simulink model "sampleModel1983"  (R2023a)
settings: Solver=VariableStepAuto  StartTime=0.0  StopTime=10.0  RelTol=1e-3
libraries: hdlsllib x7, simulink x2
settings Model: Creator=user1  LastModifiedBy=user1

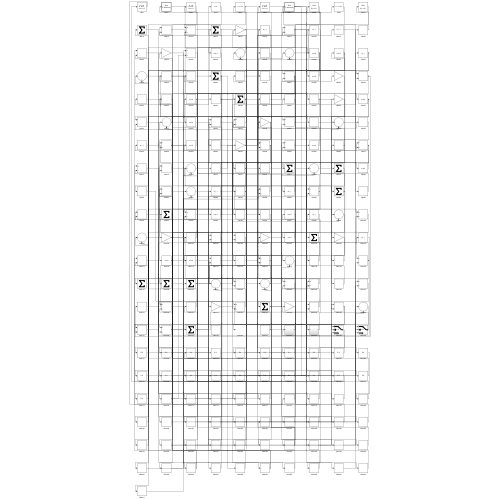
[thumbnail: Simulink's stored preview of the top-level diagram]
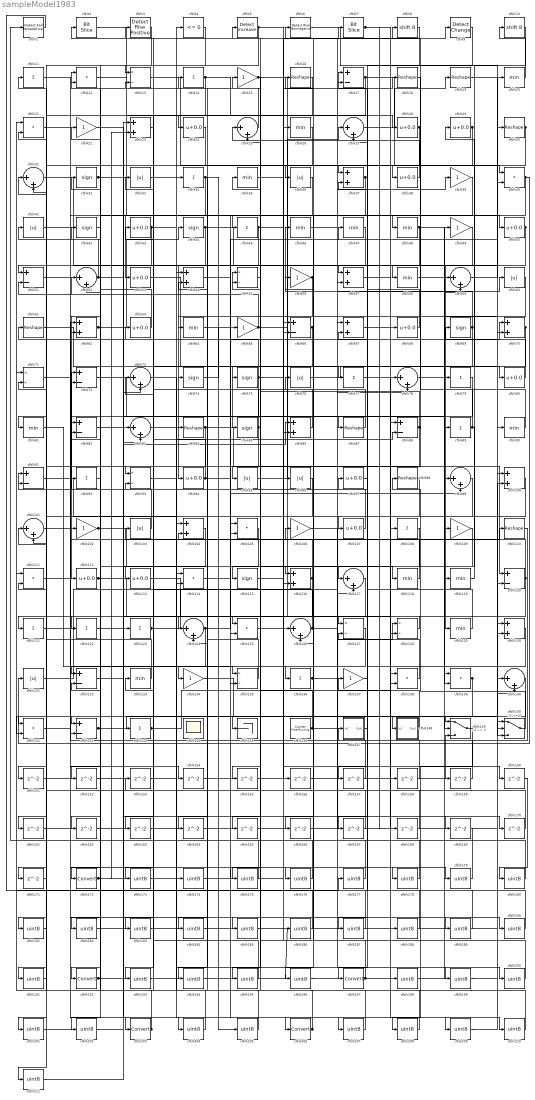
== system sampleModel1983 ==
  cfblk1 : hdlsllib/Logic and Bit Operations/Detect Fall Nonpositive  vinit=0  OutDataTypeStr=boolean
  cfblk10 : ArithShift  BitShiftNumber=8
  cfblk{23,37,54,57,62,67,70,86,100,104,116,130} (12 alike) : Sum
  cfblk{25,27,31,52,59,73,78,83,99,101,117,124,126,140} (14 alike) : Sum  Inputs=|++
  cfblk{15,22,39,49,56,65,102,106,109,134,137} (11 alike) : Gain
  cfblk{33,36,41,60,76,95..96,103,131} (9 alike) : Abs  SaturateOnIntegerOverflow=off
  cfblk{12,21,40,105,111,114,125,138..139,141} (10 alike) : DotProduct  OutDataTypeStr=Inherit: Inherit via internal rule
  cfblk{24,28..29,38,43,50,53,63,68,80,94,97,107,112..113} (15 alike) : Bias  Bias=0.0  SaturateOnIntegerOverflow=off
  cfblk{11,14,34,45,77,79,89,92,108,121..123,136,143} (14 alike) : Sum  Inputs=+
  cfblk{16,18..19,30,61,84,87,98,110} (9 alike) : Reshape
  cfblk{32,42,44,69,74..75,85,115} (8 alike) : Signum
  cfblk{20,26,35,46..48,58,64,81,90,118..119,129,133} (14 alike) : MinMax
  cfblk{17,51,66,72,82,88,91,120,132,142} (10 alike) : Sum  Inputs=+-
  cfblk{13,55,71,93,127..128,135} (7 alike) : Product  Inputs=*/  RndMeth=Zero  SaturateOnIntegerOverflow=on
  cfblk144 : Scope
      settings: Floating=on
  cfblk145 : Terminator
  cfblk146 : hdlsllib/Sources/Counter Free-Running  NumBits=16  tsamp=-1
  cfblk147 : Subsystem
      settings: LibrarySourceBlock=|
      | hdlsllib/Ports &
      | Subsystems/Subsystem
  cfblk148 : Subsystem
      settings: LibrarySourceBlock=|
      | hdlsllib/Ports &
      | Subsystems/Subsystem
  cfblk149 : Switch  SaturateOnIntegerOverflow=off  InputSameDT=off
  cfblk150 : Switch  SaturateOnIntegerOverflow=off  InputSameDT=off
  cfblk{151..171} (21 alike) : Delay  SampleTime=1
  cfblk{172,192,197,203,206} (5 alike) : DataTypeConversion  SaturateOnIntegerOverflow=off  RndMeth=Floor
  cfblk{173..191,193..196,198..202,204..205,207..211} (35 alike) : DataTypeConversion  OutDataTypeStr=uint8  SaturateOnIntegerOverflow=off  RndMeth=Floor
  cfblk2 : hdlsllib/Logic and Bit Operations/Bit Slice  lidx=7  ridx=0
  cfblk3 : hdlsllib/Logic and Bit Operations/Detect Rise Positive  vinit=0  OutDataTypeStr=boolean
  cfblk4 : hdlsllib/Logic and Bit Operations/Compare To Zero  relop=<=  OutDataTypeStr=boolean
  cfblk5 : simulink/Logic and Bit Operations/Detect Increase  vinit=0.0  OutDataTypeStr=boolean
      settings: LibrarySourceBlock=|
      | hdlsllib/Logic and Bit
      | Operations/Detect
      | Increase
  cfblk6 : hdlsllib/Logic and Bit Operations/Detect Rise Nonnegative  vinit=0  OutDataTypeStr=boolean
  cfblk7 : hdlsllib/Logic and Bit Operations/Bit Slice  lidx=7  ridx=0
  cfblk8 : ArithShift  BitShiftNumber=8
  cfblk9 : simulink/Logic and Bit Operations/Detect Change  vinit=0  OutDataTypeStr=boolean
      settings: LibrarySourceBlock=|
      | hdlsllib/Logic and Bit
      | Operations/Detect
      | Change
  wires:
  cfblk44/1 -> cfblk57/1, cfblk116/1, cfblk181/1
  cfblk33/1 -> cfblk34/1
  cfblk122/1 -> cfblk123/1
  cfblk25/1 -> cfblk12/1
  cfblk134/1 -> cfblk148/1(In1)
  cfblk38/1 -> cfblk25/1
  cfblk18/1 -> cfblk95/1
  cfblk95/1 -> cfblk27/1
  cfblk15/1 -> cfblk127/1, cfblk45/1
  cfblk4/1 -> cfblk172/1
  cfblk120/1 -> cfblk27/2, cfblk124/2
  cfblk116/1 -> cfblk3/1, cfblk201/1
  cfblk81/1 -> cfblk135/1
  cfblk86/1 -> cfblk76/1
  cfblk52/1 -> cfblk41/1, cfblk116/2
  cfblk50/1 -> cfblk94/1, cfblk139/2
  cfblk110/1 -> cfblk147/1(In1)
  cfblk74/1 -> cfblk65/1
  cfblk13/1 -> cfblk40/1
  cfblk40/1 -> cfblk131/1, cfblk59/1
  cfblk143/1 -> cfblk84/1, cfblk128/2
  cfblk8/1 -> cfblk107/1
  cfblk55/1 -> cfblk15/1
  cfblk62/1 -> cfblk44/1, cfblk86/2
  cfblk130/1 -> cfblk197/1
  cfblk42/1 -> cfblk112/1
  cfblk69/1 -> cfblk46/1, cfblk105/2
  cfblk66/1 -> cfblk163/1, cfblk164/1
  cfblk112/1 -> cfblk138/2, cfblk82/1
  cfblk36/1 -> cfblk53/1
  cfblk59/1 -> cfblk30/1
  cfblk65/1 -> cfblk20/1, cfblk8/1, cfblk51/2
  cfblk87/1 -> cfblk61/1
  cfblk3/1 -> cfblk81/1
  cfblk28/1 -> cfblk38/1, cfblk31/2, cfblk167/1
  cfblk71/1 -> cfblk203/1
  cfblk128/1 -> cfblk121/1
  cfblk94/1 -> cfblk43/1, cfblk70/1
  cfblk85/1 -> cfblk63/1, cfblk191/1
  cfblk9/1 -> cfblk37/1
  cfblk20/1 -> cfblk10/1
  cfblk68/1 -> cfblk17/1
  cfblk79/1 -> cfblk102/1
  cfblk103/1 -> cfblk11/1
  cfblk117/1 -> cfblk126/2
  cfblk118/1 -> cfblk16/1
  cfblk76/1 -> cfblk80/1
  cfblk58/1 -> cfblk129/1
  cfblk102/1 -> cfblk117/1, cfblk86/1
  cfblk131/1 -> cfblk26/1
  cfblk150/1 -> cfblk98/1
  cfblk105/1 -> cfblk115/1
  cfblk32/1 -> cfblk135/2, cfblk204/1
  cfblk56/1 -> cfblk74/1, cfblk75/1
  cfblk53/1 -> cfblk105/1
  cfblk114/1 -> cfblk47/1
  cfblk75/1 -> cfblk134/1, cfblk18/1, cfblk13/2
  cfblk133/1 -> cfblk91/1
  cfblk34/1 -> cfblk124/1, cfblk173/1, cfblk205/1
  cfblk78/1 -> cfblk89/1
  cfblk31/1 -> cfblk90/1
  cfblk17/1 -> cfblk40/2, cfblk141/1, cfblk170/1
  cfblk148/1(Out1) -> cfblk127/2
  cfblk147/1(Out1) -> cfblk37/2
  cfblk104/1 -> cfblk192/1
  cfblk39/1 -> cfblk142/1
  cfblk26/1 -> cfblk36/1
  cfblk12/1 -> cfblk108/1
  cfblk138/1 -> cfblk67/2
  cfblk124/1 -> cfblk142/2, cfblk99/2
  cfblk142/1 -> cfblk150/2, cfblk169/1
  cfblk82/1 -> cfblk125/1
  cfblk35/1 -> cfblk118/1
  cfblk126/1 -> cfblk60/1, cfblk33/1
  cfblk70/1 -> cfblk113/1, cfblk85/1
  cfblk48/1 -> cfblk132/1, cfblk70/2
  cfblk139/1 -> cfblk145/1, cfblk141/2
  cfblk41/1 -> cfblk58/1
  cfblk125/1 -> cfblk17/2
  cfblk107/1 -> cfblk72/1
  cfblk93/1 -> cfblk88/2
  cfblk43/1 -> cfblk48/1, cfblk211/1
  cfblk72/1 -> cfblk109/1
  cfblk132/1 -> cfblk143/1
  cfblk129/1 -> cfblk103/1
  cfblk108/1 -> cfblk136/1
  cfblk135/1 -> cfblk14/1
  cfblk47/1 -> cfblk64/1
  cfblk84/1 -> cfblk120/1, cfblk92/1
  cfblk14/1 -> cfblk28/1, cfblk193/1
  cfblk46/1 -> cfblk39/1
  cfblk6/1 -> cfblk150/3
  cfblk113/1 -> cfblk125/2
  cfblk64/1 -> cfblk149/1
  cfblk30/1 -> cfblk87/1, cfblk62/2
  cfblk90/1 -> cfblk7/1
  cfblk27/1 -> cfblk19/1
  cfblk11/1 -> cfblk50/1
  cfblk63/1 -> cfblk32/1
  cfblk16/1 -> cfblk24/1
  cfblk23/1 -> cfblk93/1
  cfblk88/1 -> cfblk55/1, cfblk162/1
  cfblk141/1 -> cfblk72/2
  cfblk100/1 -> cfblk122/1
  cfblk10/1 -> cfblk79/1
  cfblk29/1 -> cfblk51/1, cfblk155/1
  cfblk91/1 -> cfblk114/1
  cfblk54/1 -> cfblk206/1
  cfblk80/1 -> cfblk69/1
  cfblk5/1 -> cfblk66/2, cfblk13/1
  cfblk7/1 -> cfblk99/1, cfblk168/1, cfblk210/1
  cfblk89/1 -> cfblk119/1, cfblk2/1
  cfblk37/1 -> cfblk166/1, cfblk194/1, cfblk196/1
  cfblk61/1 -> cfblk77/1
  cfblk2/1 -> cfblk68/1
  cfblk146/1 -> cfblk149/2, cfblk25/2
  cfblk121/1 -> cfblk110/1
  cfblk45/1 -> cfblk160/1, cfblk161/1
  cfblk123/1 -> cfblk78/2, cfblk57/2
  cfblk119/1 -> cfblk29/1
  cfblk136/1 -> cfblk9/1, cfblk128/1
  cfblk19/1 -> cfblk100/1
  cfblk24/1 -> cfblk151/1
  cfblk151/1 -> cfblk114/2
  cfblk98/1 -> cfblk152/1
  cfblk51/1 -> cfblk154/1
  cfblk154/1 -> cfblk126/1
  cfblk155/1 -> cfblk149/3
  cfblk115/1 -> cfblk156/1
  cfblk97/1 -> cfblk157/1
  cfblk157/1 -> cfblk67/1
  cfblk57/1 -> cfblk158/1
  cfblk158/1 -> cfblk62/1
  cfblk159/1 -> cfblk88/1
  cfblk161/1 -> cfblk117/2
  cfblk162/1 -> cfblk59/2
  cfblk163/1 -> cfblk138/1
  cfblk164/1 -> cfblk120/2
  cfblk109/1 -> cfblk165/1
  cfblk165/1 -> cfblk78/1
  cfblk166/1 -> cfblk100/2
  cfblk167/1 -> cfblk52/2
  cfblk168/1 -> cfblk31/1
  cfblk169/1 -> cfblk1/1
  cfblk170/1 -> cfblk132/2
  cfblk96/1 -> cfblk171/1
  cfblk171/1 -> cfblk91/2
  cfblk172/1 -> cfblk96/1, cfblk23/2, cfblk52/1
  cfblk173/1 -> cfblk4/1
  cfblk153/1 -> cfblk174/1
  cfblk60/1 -> cfblk175/1
  cfblk175/1 -> cfblk153/1
  cfblk21/1 -> cfblk176/1
  cfblk176/1 -> cfblk133/1
  cfblk1/1 -> cfblk177/1
  cfblk177/1 -> cfblk21/1
  cfblk174/1 -> cfblk178/1
  cfblk178/1 -> cfblk21/2
  cfblk101/1 -> cfblk179/1
  cfblk179/1 -> cfblk23/1
  cfblk160/1 -> cfblk180/1
  cfblk180/1 -> cfblk101/1
  cfblk181/1 -> cfblk101/2
  cfblk140/1 -> cfblk182/1
  cfblk182/1 -> cfblk159/1
  cfblk99/1 -> cfblk183/1
  cfblk183/1 -> cfblk140/1
  cfblk127/1 -> cfblk184/1
  cfblk184/1 -> cfblk140/2
  cfblk22/1 -> cfblk185/1
  cfblk185/1 -> cfblk55/2
  cfblk186/1 -> cfblk22/1
  cfblk137/1 -> cfblk187/1
  cfblk187/1 -> cfblk106/1
  cfblk77/1 -> cfblk188/1
  cfblk188/1 -> cfblk137/1
  cfblk111/1 -> cfblk189/1
  cfblk189/1 -> cfblk97/1
  cfblk106/1 -> cfblk190/1
  cfblk190/1 -> cfblk111/1
  cfblk191/1 -> cfblk111/2
  cfblk192/1 -> cfblk186/1, cfblk139/1
  cfblk193/1 -> cfblk104/1
  cfblk194/1 -> cfblk104/2
  cfblk49/1 -> cfblk195/1
  cfblk195/1 -> cfblk93/2
  cfblk196/1 -> cfblk49/1
  cfblk197/1 -> cfblk56/1, cfblk6/1, cfblk35/1
  cfblk67/1 -> cfblk198/1
  cfblk198/1 -> cfblk130/1
  cfblk156/1 -> cfblk199/1
  cfblk199/1 -> cfblk130/2
  cfblk83/1 -> cfblk200/1
  cfblk200/1 -> cfblk66/1
  cfblk201/1 -> cfblk83/1
  cfblk92/1 -> cfblk202/1
  cfblk202/1 -> cfblk83/2
  cfblk203/1 -> cfblk82/2, cfblk12/2
  cfblk204/1 -> cfblk71/1
  cfblk205/1 -> cfblk71/2
  cfblk206/1 -> cfblk5/1, cfblk42/1
  cfblk152/1 -> cfblk207/1
  cfblk207/1 -> cfblk54/1
  cfblk149/1 -> cfblk208/1
  cfblk208/1 -> cfblk54/2
  cfblk73/1 -> cfblk209/1
  cfblk209/1 -> cfblk150/1
  cfblk210/1 -> cfblk73/1
  cfblk211/1 -> cfblk73/2

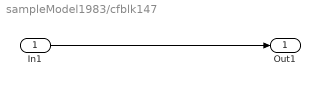
== system sampleModel1983/cfblk147 ==
  In1 : Inport
  Out1 : Outport
  wires:
  In1/1 -> Out1/1

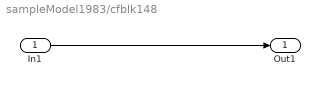
== system sampleModel1983/cfblk148 ==
  In1 : Inport
  Out1 : Outport
  wires:
  In1/1 -> Out1/1
